simulink model "cistic1"  (Simulink 7.4)
settings: Solver=ode1  StartTime=0.0  StopTime=inf  FixedStep=0.25  RelTol=1e-3  AbsTol=1e-6
libraries: simulink x4, hydro2pumps_lib x1
settings Model: Creator=dmedonza  LastModifiedBy=student
settings DataIOCC: LimitDataPoints=off  SignalLoggingName=sigsOut
settings OptimizationCC: BooleanDataType=off
settings DebuggingCC: SaveWithParameterizedLinksMsg=none  SignalResolutionControl=TryResolveAllWithWarning  SolverPrmCheckMsg=none  MultiTaskDSMMsg=warning  MultiTaskCondExecSysMsg=none  StrictBusMsg=None
settings HardwareCC: TargetUnknown=on
settings RTWCC: TemplateMakefile=grt_vc.tmf  IncludeERTFirstTime=on

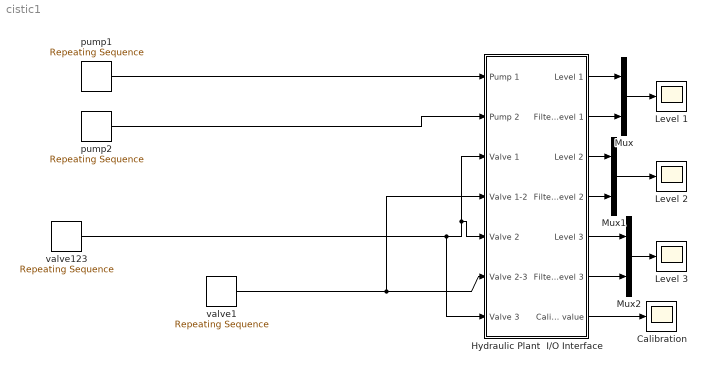
== system cistic1 ==
  Calibration : Scope
      settings: TickLabels=on  TimeRange=20  YMin=0  YMax=100  SaveName=l3nf  DataFormat=Array
  Hydraulic Plant  I/O Interface : Subsystem
      mask Display: disp('Two Pumps\nHydraulic\nPlant\nI/O Interface')
  Level 1 : Scope
      settings: TickLabels=on  TimeRange=20  YMin=2250  YMax=3100  SaveName=l1  DataFormat=Array
  Level 2 : Scope
      settings: TickLabels=on  TimeRange=20  YMin=1380  YMax=1530  SaveName=l2  DataFormat=Array
  Level 3 : Scope
      settings: TickLabels=on  TimeRange=20  YMin=2445  YMax=2470  SaveName=l3  DataFormat=Array
  Mux : Mux  Inputs=2
  Mux1 : Mux  Inputs=2
  Mux2 : Mux  Inputs=2
  pump1 : simulink/Sources/Repeating Sequence  SystemSampleTime=-1  rep_seq_t=[0 60 60 120 ]  rep_seq_y="[0 0   200 200]"
  pump2 : simulink/Sources/Repeating Sequence  SystemSampleTime=-1  rep_seq_t="[0 90  90 120]"  rep_seq_y="[0 0   200 200]"
  valve1 : simulink/Sources/Repeating Sequence  SystemSampleTime=-1  rep_seq_t=[0 2 2 4 4 6 6 8 8 60 60 120]  rep_seq_y="[1 1 0 0 1 1 0 0 1 1   1   1]"
  valve123 : simulink/Sources/Repeating Sequence  SystemSampleTime=-1  rep_seq_t=[0 2 2 4 4 6 6 8 8 60 60 120]  rep_seq_y="[1 1 0 0 1 1 0 0 1 1   0    0]"
  wires:
  Mux/1 -> Level 1/1
  Mux2/1 -> Level 3/1
  Mux1/1 -> Level 2/1
  pump1/1 -> Hydraulic Plant  I/O Interface/1(Pump 1)
  pump2/1 -> Hydraulic Plant  I/O Interface/2(Pump 2)
  valve123/1 -> Hydraulic Plant  I/O Interface/3(Valve 1), Hydraulic Plant  I/O Interface/5(Valve 2), Hydraulic Plant  I/O Interface/7(Valve 3)
  Hydraulic Plant  I/O Interface/1(Level 1) -> Mux/1
  Hydraulic Plant  I/O Interface/2(Filtered level 1) -> Mux/2
  Hydraulic Plant  I/O Interface/3(Level 2) -> Mux1/1
  Hydraulic Plant  I/O Interface/4(Filtered level 2) -> Mux1/2
  Hydraulic Plant  I/O Interface/5(Level 3) -> Mux2/1
  Hydraulic Plant  I/O Interface/6(Filtered level 3) -> Mux2/2
  Hydraulic Plant  I/O Interface/7(Calibration value) -> Calibration/1
  valve1/1 -> Hydraulic Plant  I/O Interface/6(Valve 2-3), Hydraulic Plant  I/O Interface/4(Valve 1-2)

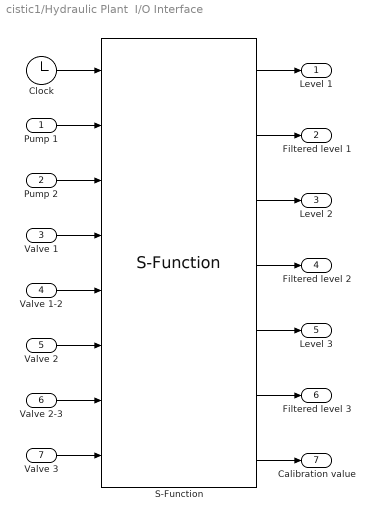
== system cistic1/Hydraulic Plant  I/O Interface ==
  Pump 1 : Inport  OutDataType=sfix(16)  OutScaling=2^0
  Pump 2 : Inport  Port=2  OutDataType=sfix(16)  OutScaling=2^0
  Valve 1 : Inport  Port=3  OutDataType=sfix(16)  OutScaling=2^0
  Valve 1-2 : Inport  Port=4  OutDataType=sfix(16)  OutScaling=2^0
  Valve 2 : Inport  Port=5  OutDataType=sfix(16)  OutScaling=2^0
  Valve 2-3 : Inport  Port=6  OutDataType=sfix(16)  OutScaling=2^0
  Valve 3 : Inport  Port=7  OutDataType=sfix(16)  OutScaling=2^0
  Clock : Clock
      settings: Decimation=10
  S-Function : hydro2pumps_lib/S-Function  Priority=1  com_port=COM4  Ts=0.25  events_ot=2  rd_timeout=125  matlab_prior=ABOVE_NORMAL_PRIORITY  warning=on  printout=off
  Level 1 : Outport
  Filtered level 1 : Outport  Port=2
  Level 2 : Outport  Port=3
  Filtered level 2 : Outport  Port=4
  Level 3 : Outport  Port=5
  Filtered level 3 : Outport  Port=6
  Calibration value : Outport  Port=7
  wires:
  S-Function/1 -> Level 1/1
  S-Function/2 -> Filtered level 1/1
  Clock/1 -> S-Function/1
  Pump 1/1 -> S-Function/2
  Pump 2/1 -> S-Function/3
  S-Function/3 -> Level 2/1
  S-Function/4 -> Filtered level 2/1
  S-Function/5 -> Level 3/1
  S-Function/6 -> Filtered level 3/1
  Valve 1/1 -> S-Function/4
  Valve 1-2/1 -> S-Function/5
  Valve 2/1 -> S-Function/6
  Valve 2-3/1 -> S-Function/7
  S-Function/7 -> Calibration value/1
  Valve 3/1 -> S-Function/8
